simulink model "final_proj_model"  (R2020b)
settings: Solver=ode23tb  StartTime=0  StopTime=365*24*60*60  RelTol=1e-4  EnableMultiTasking=on
StartFcn:
  | tic
StopFcn:
  | toc
values from neighbouring files (symbols this model uses):
  BP1 = [1:24]'    [Build_LoadProfile_Datasets.m]    (also in LoadProfile_Datasets.mat = [1 2 3 4 5 6 7 8 9 10 11 12 ... (24 elements, 24x1)])
  BP2 = [1:3]    [Build_LoadProfile_Datasets.m]    (also in LoadProfile_Datasets.mat = [1 2 3])
  BP3 = [1:2]    [Build_LoadProfile_Datasets.m]    (also in LoadProfile_Datasets.mat = [1 2])
  LoadProfile_Data = [1 2 3 4 5 6 7 8 9 10 11 12 ... (144 elements, 24x3x2)]    [LoadProfile_Datasets.mat]
undefined symbols (not defined in the file or in its folder): A, B, C, D1, Dd, Delta, j, StationData
libraries: powerlib x43, simulink x10, powerlib_meascontrol x8
(part 2 of 2)

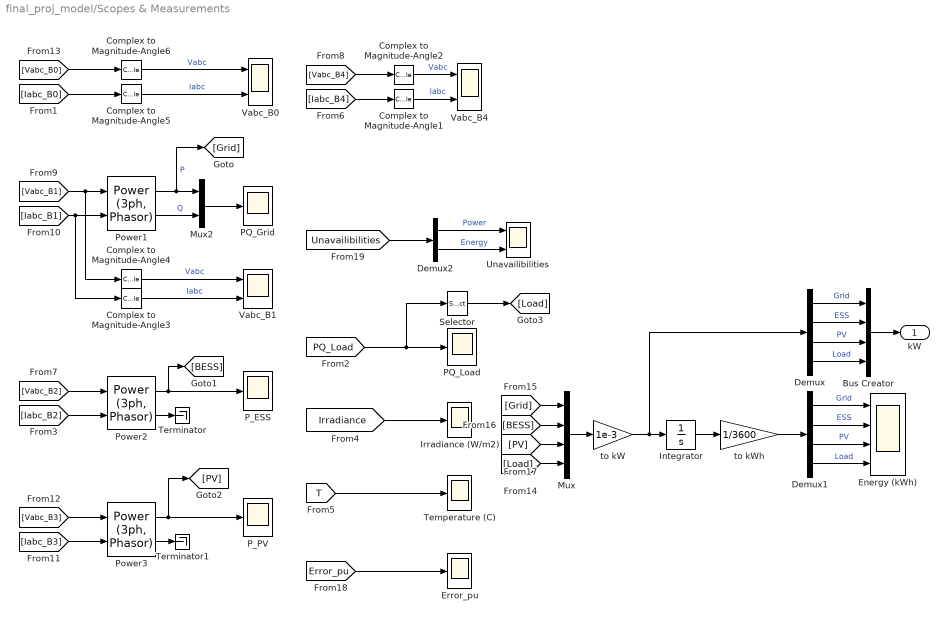
== system final_proj_model/Scopes & Measurements ==
  Bus Creator : BusCreator  Inputs=4
  Complex to Magnitude-Angle{1..6} (6 alike) : ComplexToMagnitudeAngle  Output=Magnitude
  Demux : Demux
  Demux1 : Demux
  Demux2 : Demux  Outputs=2
  Energy (kWh) : Scope  NumInputPorts=4
  Error_pu : Scope
  Integrator : Integrator
  Irradiance (W/m2) : Scope
  Mux : Mux
  Mux2 : Mux  Inputs=2
  PQ_Grid : Scope
  PQ_Load : Scope
  P_ESS : Scope
  P_PV : Scope
  Power1 : powerlib_meascontrol/Measurements/Power (3ph, Phasor)
      settings: SourceProductBaseCode=PS
  Power2 : powerlib_meascontrol/Measurements/Power (3ph, Phasor)
      settings: SourceProductBaseCode=PS
  Power3 : powerlib_meascontrol/Measurements/Power (3ph, Phasor)
      settings: SourceProductBaseCode=PS
  Selector : Selector  InputPortWidth=2  IndexOptions=Index vector (dialog)  Indices=[1]  OutputSizes=1
  Temperature (C) : Scope
  Terminator : Terminator
  Terminator1 : Terminator
  Unavailibilities : Scope  NumInputPorts=2
  Vabc_B0 : Scope  NumInputPorts=2
  Vabc_B1 : Scope  NumInputPorts=2
  Vabc_B4 : Scope  NumInputPorts=2
  to kW : Gain  Gain=1e-3
  to kWh : Gain  Gain=1/3600
  kW : Outport
  wires:
  [Iabc_B1] -> Complex to Magnitude-Angle3/1, Power1/2
  [Vabc_B1] -> Complex to Magnitude-Angle4/1, Power1/1
  Power1/1 -> [Grid], Mux2/1  "P"
  Power1/2 -> Mux2/2  "Q"
  [Iabc_B2] -> Power2/2
  [Vabc_B2] -> Power2/1
  Power2/1 -> P_ESS/1, [BESS]
  [Iabc_B3] -> Power3/2
  [Vabc_B3] -> Power3/1
  Power3/1 -> P_PV/1, [PV]
  Mux2/1 -> PQ_Grid/1
  Complex to Magnitude-Angle4/1 -> Vabc_B1/1  "Vabc"
  Complex to Magnitude-Angle3/1 -> Vabc_B1/2  "Iabc"
  Power2/2 -> Terminator/1
  Power3/2 -> Terminator1/1
  Integrator/1 -> to kWh/1
  Selector/1 -> [Load]
  Bus Creator/1 -> kW/1
  [Grid] -> Mux/1
  [PV] -> Mux/3
  [BESS] -> Mux/2
  [Load] -> Mux/4
  Mux/1 -> to kW/1
  to kW/1 -> Demux/1, Integrator/1
  to kWh/1 -> Demux1/1
  Demux/1 -> Bus Creator/1  "Grid"
  Demux/2 -> Bus Creator/2  "ESS"
  Demux/3 -> Bus Creator/3  "PV"
  Demux/4 -> Bus Creator/4  "Load"
  Demux1/1 -> Energy (kWh)/1  "Grid"
  Demux1/2 -> Energy (kWh)/2  "ESS"
  Demux1/3 -> Energy (kWh)/3  "PV"
  Demux1/4 -> Energy (kWh)/4  "Load"
  [Irradiance] -> Irradiance (W/m2)/1
  [T] -> Temperature (C)/1
  Complex to Magnitude-Angle2/1 -> Vabc_B4/1  "Vabc"
  Complex to Magnitude-Angle1/1 -> Vabc_B4/2  "Iabc"
  [Vabc_B4] -> Complex to Magnitude-Angle2/1
  [Iabc_B4] -> Complex to Magnitude-Angle1/1
  Complex to Magnitude-Angle6/1 -> Vabc_B0/1  "Vabc"
  Complex to Magnitude-Angle5/1 -> Vabc_B0/2  "Iabc"
  [Vabc_B0] -> Complex to Magnitude-Angle6/1
  [Iabc_B0] -> Complex to Magnitude-Angle5/1
  [PQ_Load] -> Selector/1, PQ_Load/1
  [Error_pu] -> Error_pu/1
  [Unavailibilities] -> Demux2/1
  Demux2/1 -> Unavailibilities/1  "Power"
  Demux2/2 -> Unavailibilities/2  "Energy"

== system final_proj_model/Subsystem ==
  Com : Inport
  Fault A : powerlib/Elements/Breaker  InitialState=0  SwitchingTimes=[1e9 1e9+1]  External=on  BreakerResistance=1e-3  SnubberResistance=1e6  SnubberCapacitance=inf  Measurements=None  MoreParameters=off  NoBreakLoop=off
  Fault A1 : powerlib/Elements/Breaker  InitialState=0  SwitchingTimes=[1e9 1e9+1]  External=on  BreakerResistance=1e-3  SnubberResistance=1e6  SnubberCapacitance=inf  Measurements=None  MoreParameters=off  NoBreakLoop=off
  Fault A2 : powerlib/Elements/Breaker  InitialState=0  SwitchingTimes=[1e9 1e9+1]  External=on  BreakerResistance=1e-3  SnubberResistance=1e6  SnubberCapacitance=inf  Measurements=None  MoreParameters=off  NoBreakLoop=off
  a : PMIOPort  Side=Right
  A : PMIOPort  Port=2  Side=Left
  b : PMIOPort  Port=3  Side=Right
  B : PMIOPort  Port=4  Side=Left
  c : PMIOPort  Port=5  Side=Right
  C : PMIOPort  Port=6  Side=Left
  wires:
  Com/1 -> Fault A2/1, Fault A1/1, Fault A/1
  connections:
  Fault A1/RConn1 -- b/RConn1
  Fault A1/LConn1 -- B/RConn1
  Fault A/LConn1 -- A/RConn1
  Fault A2/LConn1 -- C/RConn1
  Fault A/RConn1 -- a/RConn1
  Fault A2/RConn1 -- c/RConn1

== system final_proj_model/TMY3 Data ==
  note: The Irradiance table data are stored in the .mat file StationData_NEW.
      | This file is loaded at  mask initialization.
  note: TMY3 (Typical Meterological Year) files have been produced by NREL's
      | Electric Systems Center under the Solar Resource Characterization Project,
      | which is funded and monitored by the U.S. Department of Energy's Energy
      |  Efficiency and Renewable Energy Office.
  note: National Renewable Energy Laboratory
      | 1617 Cole Boulevard, Golden, Colorado 80401-3393
      | 303-275-3000  www.nrel.gov
  note: Reference: Users Manual for TMY3 Data Sets
      | S. Wilcox and W. Marion
  note: Definition:
      |
      | Global horizontal irradiance, Watt-hour per square meter (Wh/m2)
      | Total amount of direct and diffuse solar radiation received on a
      | horizontal surface during the 60-minute period ending at the timestamp.
      |
      | Diffuse horizontal irradiance, Watt-hour per square meter (Wh/m2)
      | Amount of solar radiation received from the sky (excluding the solar disk)
      | on a horizontal surface during the 60-minute period ending at the timestamp.
      |
      | Direct normal irradiance, Watt-hour per square meter (Wh/m2)
      | Amount of solar radiation (modeled) received in a collimated beam on a surface
      | normal to the sun during the 60-minute period ending at the timestamp.
  1-D Lookup IRRADIANCE Table : Lookup_n-D  NumberOfTableDimensions=1  BreakpointsForDimension1=[1:size(StationData(Index).Temperature,1)]  Table=IrradianceTable  InterpMethod=Flat  InternalRulePriority=Speed  RndMeth=Simplest  InputSameDT=on
  1-D Lookup TEMPERATURE (C) Table : Lookup_n-D  NumberOfTableDimensions=1  BreakpointsForDimension1=[1:size(StationData(Index).Temperature,1)]  Table=StationData(Index).Temperature  InterpMethod=Flat  InternalRulePriority=Speed  RndMeth=Simplest  InputSameDT=on
  1-min Filter : TransferFcn  Denominator=[60 1]
  Add : Sum
  Clock : Clock
  Constant : Constant
  Second-->Hour : Gain  Gain=1/(60*60)
  efficiency : Gain  Gain=Efficiency/100
  m2 : Gain  Gain=TotalArea
  P : Outport
  tag scope: Irradiance=global, T=global
  wires:
  m2/1 -> efficiency/1
  1-D Lookup IRRADIANCE Table/1 -> 1-min Filter/1
  Clock/1 -> Second-->Hour/1
  1-D Lookup TEMPERATURE (C) Table/1 -> [T]
  1-min Filter/1 -> [Irradiance], m2/1
  efficiency/1 -> P/1
  Constant/1 -> Add/2
  Second-->Hour/1 -> Add/1
  Add/1 -> 1-D Lookup TEMPERATURE (C) Table/1, 1-D Lookup IRRADIANCE Table/1  "Hour of the year"

== system final_proj_model/Day Of The Year/Counter ==
  Enable : EnablePort
  Add : Sum
  Constant : Constant
  Memory : Memory
  Out1 : Outport
  wires:
  Add/1 -> Out1/1, Memory/1
  Memory/1 -> Add/1
  Constant/1 -> Add/2

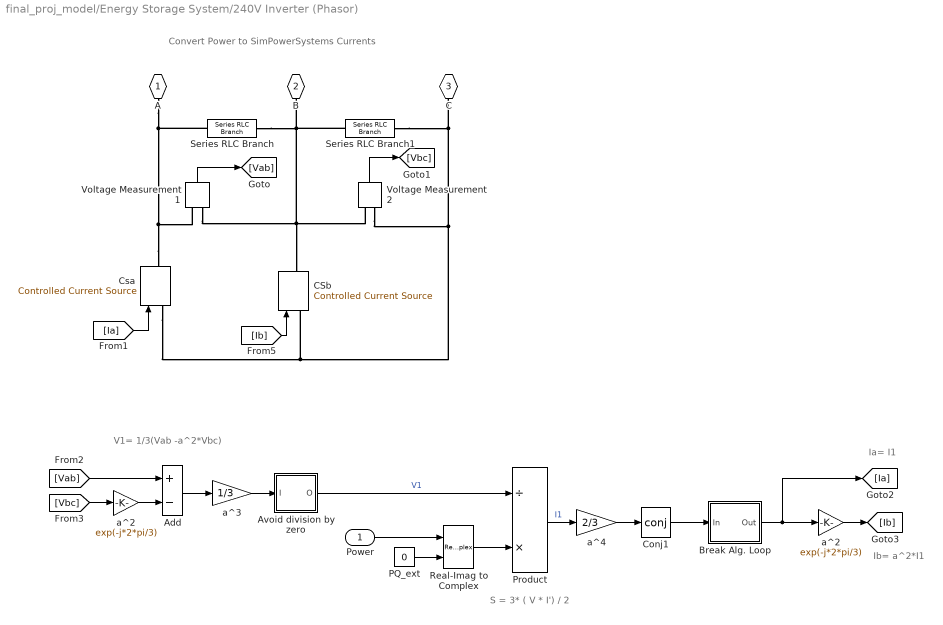
== system final_proj_model/Energy Storage System/240V Inverter (Phasor) ==
  note: V1= 1/3(Vab -a^2*Vbc)
  note: S = 3* ( V * I') / 2
  note: Ia= I1
  note: Ib= a^2*I1
  note: Convert Power to SimPowerSystems Currents
  Power : Inport
  Add : Sum  Inputs=+-
  Avoid division by zero : Subsystem
  "Break Alg. Loop " : Subsystem
  CSb : powerlib/Electrical Sources/Controlled Current Source  Initialize=off  Source_Type=AC  Amplitude=0  Phase=0  Frequency=0  Measurements=None
  Conj1 : Math  Operator=conj  SignedPower=on  SaturateOnIntegerOverflow=on
  Csa : powerlib/Electrical Sources/Controlled Current Source  Initialize=off  Source_Type=AC  Amplitude=0  Phase=0  Frequency=0  Measurements=None
  PQ_ext : Constant  Value=0
  Product : Product  Inputs=/*  InputSameDT=on  SaturateOnIntegerOverflow=on  OutDataTypeStr=Inherit: Same as first input
  Real-Imag to Complex : RealImagToComplex
  Series RLC Branch : powerlib/Elements/Series RLC Branch  LConnTagsString=__new0  RConnTagsString=__new0  BranchType=R  Resistance=1e6  Inductance=1e-3  SetiL0=off  InitialCurrent=0  Capacitance=1e-6  Setx0=off  InitialVoltage=0  Measurements=None
  Series RLC Branch1 : powerlib/Elements/Series RLC Branch  LConnTagsString=__new0  RConnTagsString=__new0  BranchType=R  Resistance=1e6  Inductance=1e-3  SetiL0=off  InitialCurrent=0  Capacitance=1e-6  Setx0=off  InitialVoltage=0  Measurements=None
  Voltage Measurement1 : powerlib/Measurements/Voltage Measurement  PhasorSimulation=on  OutputType=Complex  PSBequivalent=0
  Voltage Measurement2 : powerlib/Measurements/Voltage Measurement  PhasorSimulation=on  OutputType=Complex  PSBequivalent=0
  a^2 : Gain  Gain=exp(-j*2*pi/3)  SaturateOnIntegerOverflow=on  OutDataTypeStr=Inherit: Same as input  ParamDataTypeStr=Inherit: Same as input
  "a^2 " : Gain  Gain=exp(-j*2*pi/3)  SaturateOnIntegerOverflow=on  OutDataTypeStr=Inherit: Same as input  ParamDataTypeStr=Inherit: Same as input
  a^3 : Gain  Gain=1/3  SaturateOnIntegerOverflow=on  OutDataTypeStr=Inherit: Same as input  ParamDataTypeStr=Inherit: Same as input
  a^4 : Gain  Gain=2/3  SaturateOnIntegerOverflow=on  OutDataTypeStr=Inherit: Same as input  ParamDataTypeStr=Inherit: Same as input
  A : PMIOPort  Tag=PMCPort  Side=Right
  B : PMIOPort  Tag=PMCPort  Port=2  Side=Right
  C : PMIOPort  Tag=PMCPort  Port=3  Side=Right
  wires:
  Power/1 -> Real-Imag to Complex/1
  Real-Imag to Complex/1 -> Product/2
  Product/1 -> a^4/1  "I1"
  PQ_ext/1 -> Real-Imag to Complex/2
  a^2/1 -> [Ib]
  Avoid division by zero/1(O) -> Product/1  "V1"
  Conj1/1 -> "Break Alg. Loop "/1(In)
  a^3/1 -> Avoid division by zero/1(I)
  Add/1 -> a^3/1
  [Vab] -> Add/1
  [Vbc] -> "a^2 "/1
  "a^2 "/1 -> Add/2
  a^4/1 -> Conj1/1
  "Break Alg. Loop "/1(Out) -> [Ia], a^2/1
  [Ib] -> CSb/1
  [Ia] -> Csa/1
  Voltage Measurement2/1 -> [Vbc]
  Voltage Measurement1/1 -> [Vab]
  connections:
  Series RLC Branch/RConn1 -- B/RConn1 -- Series RLC Branch1/LConn1 -- CSb/RConn1 -- Voltage Measurement1/LConn2 -- Voltage Measurement2/LConn1
  Series RLC Branch1/RConn1 -- C/RConn1 -- Csa/LConn1 -- CSb/LConn1 -- Voltage Measurement2/LConn2
  Csa/RConn1 -- A/RConn1 -- Series RLC Branch/LConn1 -- Voltage Measurement1/LConn1

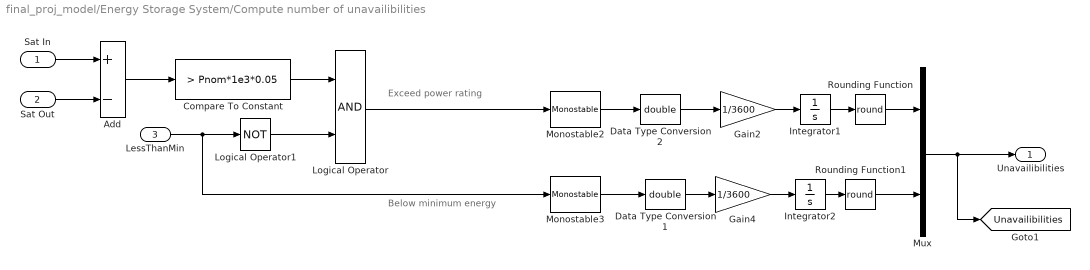
== system final_proj_model/Energy Storage System/Compute number of unavailibilities ==
  note: Exceed power rating
  note: Below minimum energy
  Sat In : Inport
  Sat Out : Inport  Port=2
  LessThanMin : Inport  Port=3
  Add : Sum  Inputs=+-
  Compare To Constant : simulink/Logic and Bit Operations/Compare To Constant  relop=>  const=Pnom*1e3*0.05  OutDataTypeStr=uint8
  Data Type Conversion1 : DataTypeConversion  OutDataTypeStr=double
  Data Type Conversion2 : DataTypeConversion  OutDataTypeStr=double
  Gain2 : Gain  Gain=1/3600
  Gain4 : Gain  Gain=1/3600
  Integrator1 : Integrator
  Integrator2 : Integrator
  Logical Operator : Logic  AllPortsSameDT=off  OutDataTypeStr=boolean
  Logical Operator1 : Logic  Operator=NOT  AllPortsSameDT=off  OutDataTypeStr=boolean
  Monostable2 : powerlib_meascontrol/Logic/Monostable  EdgeDetect=Rising  PulseDuration=3600  ic=0  Ts=0
      settings: SourceProductBaseCode=PS
  Monostable3 : powerlib_meascontrol/Logic/Monostable  EdgeDetect=Rising  PulseDuration=3600  ic=0  Ts=0
      settings: SourceProductBaseCode=PS
  Mux : Mux  Inputs=2
  Rounding Function : Rounding  Operator=round
  Rounding Function1 : Rounding  Operator=round
  Unavailibilities : Outport
  tag scope: Unavailibilities=global
  wires:
  Add/1 -> Compare To Constant/1
  Monostable3/1 -> Data Type Conversion1/1
  Monostable2/1 -> Data Type Conversion2/1
  Data Type Conversion1/1 -> Gain4/1
  Compare To Constant/1 -> Logical Operator/1
  LessThanMin/1 -> Monostable3/1, Logical Operator1/1
  Logical Operator1/1 -> Logical Operator/2
  Data Type Conversion2/1 -> Gain2/1
  Integrator1/1 -> Rounding Function/1
  Integrator2/1 -> Rounding Function1/1
  Rounding Function/1 -> Mux/1
  Rounding Function1/1 -> Mux/2
  Mux/1 -> Unavailibilities/1, [Unavailibilities]
  Logical Operator/1 -> Monostable2/1
  Gain2/1 -> Integrator1/1
  Gain4/1 -> Integrator2/1
  Sat In/1 -> Add/1
  Sat Out/1 -> Add/2

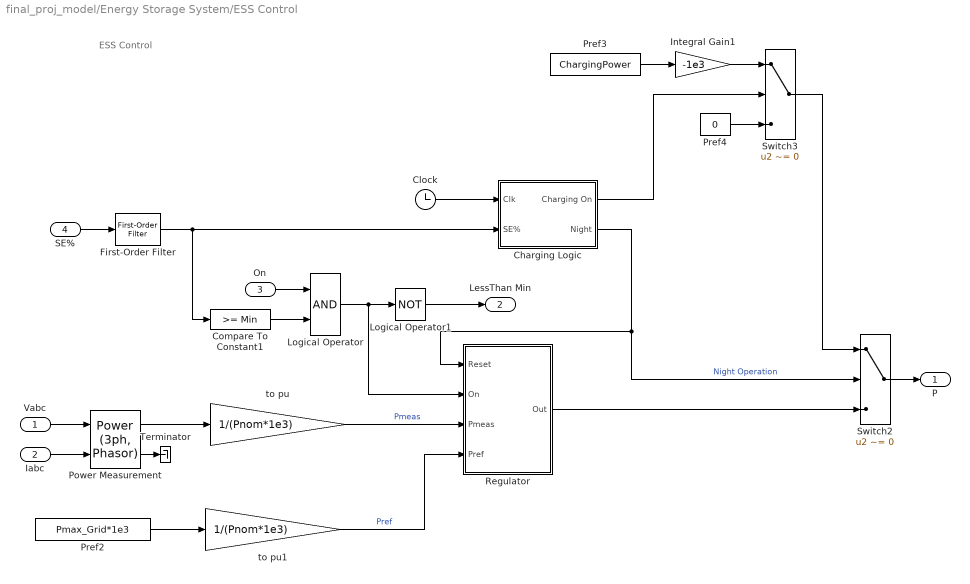
== system final_proj_model/Energy Storage System/ESS Control ==
  note: ESS Control
  Vabc : Inport
  Iabc : Inport  Port=2
  On : Inport  Port=3
  SE% : Inport  Port=4
  Charging Logic : Subsystem
  Clock : Clock
  Compare To Constant1 : simulink/Logic and Bit Operations/Compare To Constant  relop=>=  const=Min  OutDataTypeStr=boolean
  First-Order Filter : powerlib_meascontrol/Filters/First-Order Filter  FilterType=Lowpass  Tc=1  Ts=0  Initialize=on  Vac_Init=[0, 0, 60]  Vdc_Init=Max  PlotResponse=off  FreqRange="[0,  200,  1]"
  Integral Gain1 : Gain  Gain=-1e3
  Logical Operator : Logic  AllPortsSameDT=off  OutDataTypeStr=boolean
  Logical Operator1 : Logic  Operator=NOT  AllPortsSameDT=off  OutDataTypeStr=boolean
  Power Measurement : powerlib_meascontrol/Measurements/Power (3ph, Phasor)
      settings: SourceProductBaseCode=PS
  Pref2 : Constant  Value=Pmax_Grid*1e3
  Pref3 : Constant  Value=ChargingPower
  Pref4 : Constant  Value=0
  Regulator : Subsystem
  Switch2 : Switch  Criteria=u2 ~= 0  Threshold=0.5
  Switch3 : Switch  Criteria=u2 ~= 0  Threshold=0.5
  Terminator : Terminator
  to pu : Gain  Gain=1/(Pnom*1e3)
  to pu1 : Gain  Gain=1/(Pnom*1e3)
  P : Outport  OutputWhenDisabled=reset  InitialOutput=0
  LessThan Min : Outport  Port=2  OutputWhenDisabled=reset  InitialOutput=0
  wires:
  Power Measurement/2 -> Terminator/1
  Vabc/1 -> Power Measurement/1
  Iabc/1 -> Power Measurement/2
  Power Measurement/1 -> to pu/1
  Compare To Constant1/1 -> Logical Operator/2
  SE%/1 -> First-Order Filter/1
  Switch2/1 -> P/1
  Pref3/1 -> Integral Gain1/1
  On/1 -> Logical Operator/1
  Clock/1 -> Charging Logic/1(Clk)
  First-Order Filter/1 -> Compare To Constant1/1, Charging Logic/2(SE%)
  Logical Operator/1 -> Regulator/2(On), Logical Operator1/1
  Pref2/1 -> to pu1/1
  Logical Operator1/1 -> LessThan Min/1
  Integral Gain1/1 -> Switch3/1
  Pref4/1 -> Switch3/3
  Switch3/1 -> Switch2/1
  Charging Logic/2(Night) -> Regulator/1(Reset), Switch2/2  "Night Operation"
  Charging Logic/1(Charging On) -> Switch3/2
  to pu/1 -> Regulator/3(Pmeas)  "Pmeas"
  to pu1/1 -> Regulator/4(Pref)  "Pref"
  Regulator/1(Out) -> Switch2/3

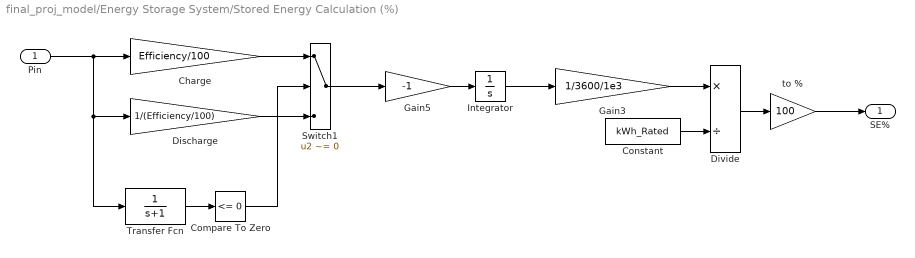
== system final_proj_model/Energy Storage System/Stored Energy Calculation (%) ==
  Pin : Inport
  Charge : Gain  Gain=Efficiency/100
  Compare To Zero : simulink/Logic and Bit Operations/Compare To Zero  relop=<=  OutDataTypeStr=boolean
  Constant : Constant  Value=kWh_Rated
  Discharge : Gain  Gain=1/(Efficiency/100)
  Divide : Product  Inputs=*/
  Gain3 : Gain  Gain=1/3600/1e3
  Gain5 : Gain  Gain=-1
  Integrator : Integrator  InitialCondition=(Initial_kWh_pc/100)*kWh_Rated*3600*1e3
  Switch1 : Switch  Criteria=u2 ~= 0
  Transfer Fcn : TransferFcn  Denominator=[1 1]
  to % : Gain  Gain=100
  SE% : Outport
  wires:
  Pin/1 -> Charge/1, Discharge/1, Transfer Fcn/1
  Integrator/1 -> Gain3/1
  Compare To Zero/1 -> Switch1/2
  Divide/1 -> to %/1
  Charge/1 -> Switch1/1
  Constant/1 -> Divide/2
  Gain3/1 -> Divide/1
  Switch1/1 -> Gain5/1
  Transfer Fcn/1 -> Compare To Zero/1
  to %/1 -> SE%/1
  Gain5/1 -> Integrator/1
  Discharge/1 -> Switch1/3

== system final_proj_model/PV Farm/Avoid division by zero ==
  I : Inport
  Complex to Magnitude-Angle : ComplexToMagnitudeAngle
  Magnitude-Angle to Complex : MagnitudeAngleToComplex
  Saturation1 : Saturate  UpperLimit=inf  LowerLimit=1e-6
  O : Outport
  wires:
  Complex to Magnitude-Angle/2 -> Magnitude-Angle to Complex/2
  Magnitude-Angle to Complex/1 -> O/1
  Complex to Magnitude-Angle/1 -> Saturation1/1
  Saturation1/1 -> Magnitude-Angle to Complex/1
  I/1 -> Complex to Magnitude-Angle/1

== system final_proj_model/PV Farm/Break Alg. Loop  ==
  In : Inport
  Complex to Real-Imag : ComplexToRealImag
  Real-Imag to Complex : RealImagToComplex
  imag : Subsystem  mask(Transfer Function with Initial Outputs){N=[1], D=[1  1], Y0=0, U0=0}
      mask prompts: N "Numerator:"; D "Denominator:"; Y0 "Initial output:"; U0 "Initial input:"
      mask help: Vector expressions for numerator, and denominator. Coefficients are in descending powers of s.
      mask init:
      | [A,B,C,Dd]=tf2ss(N,D);if (isempty(Y0));[m,n]=size(A);X0=zeros(1,m); end; if (isempty(U0));[m,p]=size(B);U0=zeros(1,p);end;X0=getxo(A,B,C,Dd,U0,Y0,0);
      mask Help: Specify the initial output for the transfer function.  An optimization routine attempts to determine the appropriate initial states so that the specified initial output is achieved.  For more details, see the m-file getxo.m
      mask Display: dpoly(N,D,'s')
  real : Subsystem  mask(Transfer Function with Initial Outputs){N=[1], D=[1  1], Y0=0, U0=0}
      mask prompts: N "Numerator:"; D "Denominator:"; Y0 "Initial output:"; U0 "Initial input:"
      mask help: Vector expressions for numerator, and denominator. Coefficients are in descending powers of s.
      mask init:
      | [A,B,C,Dd]=tf2ss(N,D);if (isempty(Y0));[m,n]=size(A);X0=zeros(1,m); end; if (isempty(U0));[m,p]=size(B);U0=zeros(1,p);end;X0=getxo(A,B,C,Dd,U0,Y0,0);
      mask Help: Specify the initial output for the transfer function.  An optimization routine attempts to determine the appropriate initial states so that the specified initial output is achieved.  For more details, see the m-file getxo.m
      mask Display: dpoly(N,D,'s')
  Out : Outport
  wires:
  imag/1(Out1) -> Real-Imag to Complex/2
  Complex to Real-Imag/2 -> imag/1(In1)
  real/1(Out1) -> Real-Imag to Complex/1
  Complex to Real-Imag/1 -> real/1(In1)
  Real-Imag to Complex/1 -> Out/1
  In/1 -> Complex to Real-Imag/1

== system final_proj_model/Residential Load/Determine Season ==
  note: Winter = First 3 months + last 3 months
  Clk : Inport
  3 months in seconds : simulink/Logic and Bit Operations/Compare To Constant  relop=>=  const=(8760*1/4)*60*60  OutDataTypeStr=boolean
  9 months in seconds : simulink/Logic and Bit Operations/Compare To Constant  relop=<  const=(8760*3/4)*60*60  OutDataTypeStr=boolean
  Logical Operator : Logic  AllPortsSameDT=off  OutDataTypeStr=boolean
  Summer : Constant  Value=2
  Switch : Switch  Criteria=u2 ~= 0
  Winter : Constant  Value=3
  Season : Outport
  wires:
  Switch/1 -> Season/1
  Clk/1 -> 9 months in seconds/1, 3 months in seconds/1
  Logical Operator/1 -> Switch/2
  Winter/1 -> Switch/3
  Summer/1 -> Switch/1
  9 months in seconds/1 -> Logical Operator/2
  3 months in seconds/1 -> Logical Operator/1

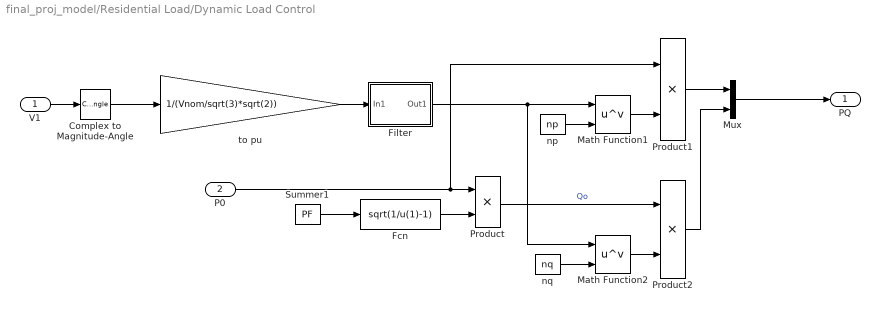
== system final_proj_model/Residential Load/Dynamic Load Control ==
  V1 : Inport
  P0 : Inport  Port=2
  Complex to Magnitude-Angle : ComplexToMagnitudeAngle  Output=Magnitude
  Fcn : Fcn  Expr=sqrt(1/u(1)-1)
  Filter : Subsystem  mask(Transfer Function with Initial Outputs){N=[1], D=[1  1], Y0=0, U0=0}
      mask prompts: N "Numerator:"; D "Denominator:"; Y0 "Initial output:"; U0 "Initial input:"
      mask help: Vector expressions for numerator, and denominator. Coefficients are in descending powers of s.
      mask init:
      | [A,B,C,Dd]=tf2ss(N,D);if (isempty(Y0));[m,n]=size(A);X0=zeros(1,m); end; if (isempty(U0));[m,p]=size(B);U0=zeros(1,p);end;X0=getxo(A,B,C,Dd,U0,Y0,0);
      mask Help: Specify the initial output for the transfer function.  An optimization routine attempts to determine the appropriate initial states so that the specified initial output is achieved.  For more details, see the m-file getxo.m
      mask Display: dpoly(N,D,'s')
  Math Function1 : Math  Operator=pow  SignedPower=on  SaturateOnIntegerOverflow=on
  Math Function2 : Math  Operator=pow  SignedPower=on  SaturateOnIntegerOverflow=on
  Mux : Mux  Inputs=2
  Product : Product
  Product1 : Product
  Product2 : Product
  Summer1 : Constant  Value=PF
  np : Constant  Value=np
  nq : Constant  Value=nq
  to pu : Gain  Gain=1/(Vnom/sqrt(3)*sqrt(2))  SaturateOnIntegerOverflow=on  OutDataTypeStr=Inherit: Same as input  ParamDataTypeStr=Inherit: Same as input
  PQ : Outport
  wires:
  Summer1/1 -> Fcn/1
  P0/1 -> Product1/1, Product/1
  Complex to Magnitude-Angle/1 -> to pu/1
  to pu/1 -> Filter/1(In1)
  Fcn/1 -> Product/2
  Product1/1 -> Mux/1
  Product2/1 -> Mux/2
  Mux/1 -> PQ/1
  Filter/1(Out1) -> Math Function2/1, Math Function1/1
  Math Function1/1 -> Product1/2
  Product/1 -> Product2/1  "Qo"
  Math Function2/1 -> Product2/2
  nq/1 -> Math Function2/2
  np/1 -> Math Function1/2
  V1/1 -> Complex to Magnitude-Angle/1

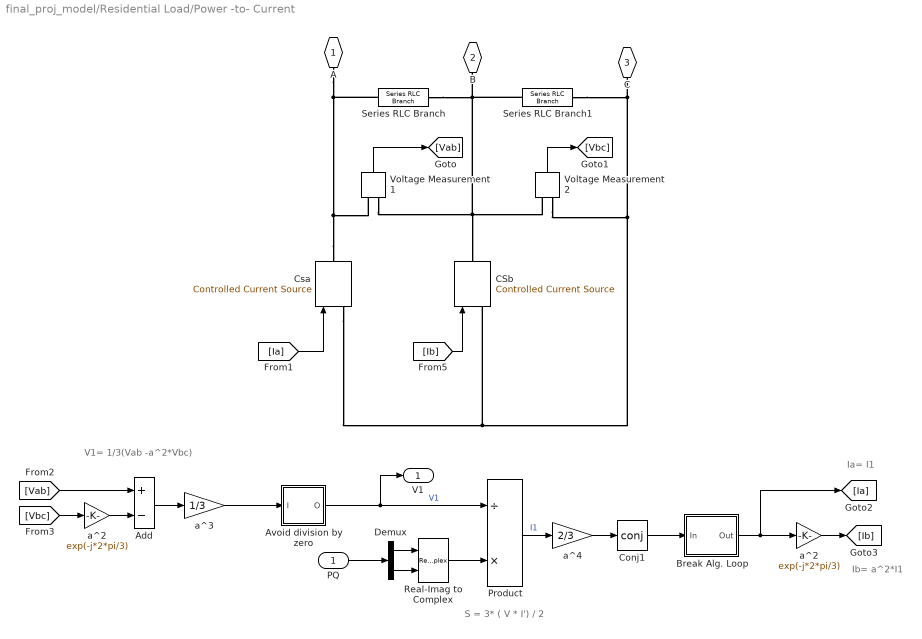
== system final_proj_model/Residential Load/Power -to- Current ==
  note: V1= 1/3(Vab -a^2*Vbc)
  note: S = 3* ( V * I') / 2
  note: Ia= I1
  note: Ib= a^2*I1
  PQ : Inport
  Add : Sum  Inputs=+-
  Avoid division by zero : Subsystem
  "Break Alg. Loop " : Subsystem
  CSb : powerlib/Electrical Sources/Controlled Current Source  Initialize=off  Source_Type=AC  Amplitude=0  Phase=0  Frequency=0  Measurements=None
  Conj1 : Math  Operator=conj  SignedPower=on  SaturateOnIntegerOverflow=on
  Csa : powerlib/Electrical Sources/Controlled Current Source  Initialize=off  Source_Type=AC  Amplitude=0  Phase=0  Frequency=0  Measurements=None
  Demux : Demux  Outputs=2
  Product : Product  Inputs=/*  InputSameDT=on  SaturateOnIntegerOverflow=on  OutDataTypeStr=Inherit: Same as first input
  Real-Imag to Complex : RealImagToComplex
  Series RLC Branch : powerlib/Elements/Series RLC Branch  LConnTagsString=__new0  RConnTagsString=__new0  BranchType=R  Resistance=1e6  Inductance=1e-3  SetiL0=off  InitialCurrent=0  Capacitance=1e-6  Setx0=off  InitialVoltage=0  Measurements=None
  Series RLC Branch1 : powerlib/Elements/Series RLC Branch  LConnTagsString=__new0  RConnTagsString=__new0  BranchType=R  Resistance=1e6  Inductance=1e-3  SetiL0=off  InitialCurrent=0  Capacitance=1e-6  Setx0=off  InitialVoltage=0  Measurements=None
  Voltage Measurement1 : powerlib/Measurements/Voltage Measurement  PhasorSimulation=on  OutputType=Complex  PSBequivalent=0
  Voltage Measurement2 : powerlib/Measurements/Voltage Measurement  PhasorSimulation=on  OutputType=Complex  PSBequivalent=0
  a^2 : Gain  Gain=exp(-j*2*pi/3)  SaturateOnIntegerOverflow=on  OutDataTypeStr=Inherit: Same as input  ParamDataTypeStr=Inherit: Same as input
  "a^2 " : Gain  Gain=exp(-j*2*pi/3)  SaturateOnIntegerOverflow=on  OutDataTypeStr=Inherit: Same as input  ParamDataTypeStr=Inherit: Same as input
  a^3 : Gain  Gain=1/3  SaturateOnIntegerOverflow=on  OutDataTypeStr=Inherit: Same as input  ParamDataTypeStr=Inherit: Same as input
  a^4 : Gain  Gain=2/3  SaturateOnIntegerOverflow=on  OutDataTypeStr=Inherit: Same as input  ParamDataTypeStr=Inherit: Same as input
  A : PMIOPort  Tag=PMCPort  Side=Right
  B : PMIOPort  Tag=PMCPort  Port=2  Side=Right
  C : PMIOPort  Tag=PMCPort  Port=3  Side=Right
  V1 : Outport
  wires:
  Voltage Measurement1/1 -> [Vab]
  Voltage Measurement2/1 -> [Vbc]
  Real-Imag to Complex/1 -> Product/2
  Product/1 -> a^4/1  "I1"
  [Ia] -> Csa/1
  a^2/1 -> [Ib]
  Avoid division by zero/1(O) -> V1/1, Product/1  "V1"
  Conj1/1 -> "Break Alg. Loop "/1(In)
  a^3/1 -> Avoid division by zero/1(I)
  Add/1 -> a^3/1
  [Vab] -> Add/1
  [Vbc] -> "a^2 "/1
  "a^2 "/1 -> Add/2
  a^4/1 -> Conj1/1
  "Break Alg. Loop "/1(Out) -> [Ia], a^2/1
  [Ib] -> CSb/1
  Demux/1 -> Real-Imag to Complex/1
  Demux/2 -> Real-Imag to Complex/2
  PQ/1 -> Demux/1
  connections:
  Csa/RConn1 -- Voltage Measurement1/LConn1 -- Series RLC Branch/LConn1 -- A/RConn1
  C/RConn1 -- Series RLC Branch1/RConn1 -- Csa/LConn1 -- CSb/LConn1 -- Voltage Measurement2/LConn2
  B/RConn1 -- Series RLC Branch/RConn1 -- Series RLC Branch1/LConn1 -- Voltage Measurement2/LConn1 -- Voltage Measurement1/LConn2 -- CSb/RConn1

== system final_proj_model/Energy Storage System/240V Inverter (Phasor)/Avoid division by zero ==
  I : Inport
  Complex to Magnitude-Angle : ComplexToMagnitudeAngle
  Magnitude-Angle to Complex : MagnitudeAngleToComplex
  Saturation1 : Saturate  UpperLimit=inf  LowerLimit=1e-6
  O : Outport
  wires:
  I/1 -> Complex to Magnitude-Angle/1
  Saturation1/1 -> Magnitude-Angle to Complex/1
  Complex to Magnitude-Angle/1 -> Saturation1/1
  Magnitude-Angle to Complex/1 -> O/1
  Complex to Magnitude-Angle/2 -> Magnitude-Angle to Complex/2

== system final_proj_model/Energy Storage System/240V Inverter (Phasor)/Break Alg. Loop  ==
  In : Inport
  Complex to Real-Imag : ComplexToRealImag
  Real-Imag to Complex : RealImagToComplex
  imag : Subsystem  mask(Transfer Function with Initial Outputs){N=[1], D=[1  1], Y0=0, U0=0}
      mask prompts: N "Numerator:"; D "Denominator:"; Y0 "Initial output:"; U0 "Initial input:"
      mask help: Vector expressions for numerator, and denominator. Coefficients are in descending powers of s.
      mask init:
      | [A,B,C,Dd]=tf2ss(N,D);if (isempty(Y0));[m,n]=size(A);X0=zeros(1,m); end; if (isempty(U0));[m,p]=size(B);U0=zeros(1,p);end;X0=getxo(A,B,C,Dd,U0,Y0,0);
      mask Help: Specify the initial output for the transfer function.  An optimization routine attempts to determine the appropriate initial states so that the specified initial output is achieved.  For more details, see the m-file getxo.m
      mask Display: dpoly(N,D,'s')
  real : Subsystem  mask(Transfer Function with Initial Outputs){N=[1], D=[1  1], Y0=0, U0=0}
      mask prompts: N "Numerator:"; D "Denominator:"; Y0 "Initial output:"; U0 "Initial input:"
      mask help: Vector expressions for numerator, and denominator. Coefficients are in descending powers of s.
      mask init:
      | [A,B,C,Dd]=tf2ss(N,D);if (isempty(Y0));[m,n]=size(A);X0=zeros(1,m); end; if (isempty(U0));[m,p]=size(B);U0=zeros(1,p);end;X0=getxo(A,B,C,Dd,U0,Y0,0);
      mask Help: Specify the initial output for the transfer function.  An optimization routine attempts to determine the appropriate initial states so that the specified initial output is achieved.  For more details, see the m-file getxo.m
      mask Display: dpoly(N,D,'s')
  Out : Outport
  wires:
  In/1 -> Complex to Real-Imag/1
  Real-Imag to Complex/1 -> Out/1
  Complex to Real-Imag/1 -> real/1(In1)
  real/1(Out1) -> Real-Imag to Complex/1
  Complex to Real-Imag/2 -> imag/1(In1)
  imag/1(Out1) -> Real-Imag to Complex/2

== system final_proj_model/Energy Storage System/ESS Control/Charging Logic ==
  note: Charging is allowed between midnight and 6 o'clock in the morning if Stored Energy is less than 90 %
  Clk : Inport
  SE% : Inport  Port=2
  1 day in hours : Constant  Value=24
  Compare To Constant : simulink/Logic and Bit Operations/Compare To Constant  relop=<  const=Max  OutDataTypeStr=boolean
  Logical Operator1 : Logic  AllPortsSameDT=off  OutDataTypeStr=boolean
  Math Function : Math  Operator=mod  SignedPower=on  SaturateOnIntegerOverflow=on
  Second-->Hour : Gain  Gain=1/(60*60)
  night : simulink/Logic and Bit Operations/Compare To Constant  relop=<  const=6  OutDataTypeStr=boolean
  Charging On : Outport
  Night : Outport  Port=2
  wires:
  Logical Operator1/1 -> Charging On/1
  Second-->Hour/1 -> Math Function/1
  Math Function/1 -> night/1
  1 day in hours/1 -> Math Function/2
  night/1 -> Night/1, Logical Operator1/1
  SE%/1 -> Compare To Constant/1
  Compare To Constant/1 -> Logical Operator1/2
  Clk/1 -> Second-->Hour/1

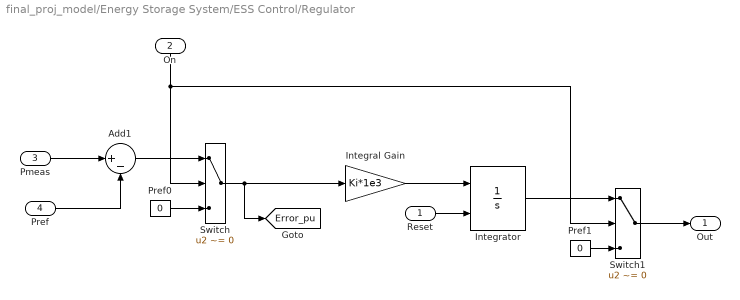
== system final_proj_model/Energy Storage System/ESS Control/Regulator ==
  Reset : Inport
  On : Inport  Port=2
  Pmeas : Inport  Port=3
  Pref : Inport  Port=4
  Add1 : Sum  Inputs=|+-
  Integral Gain : Gain  Gain=Ki*1e3
  Integrator : Integrator  ExternalReset=falling  LimitOutput=on  UpperSaturationLimit=Plimit*1.1  LowerSaturationLimit=0
  Pref0 : Constant  Value=0
  Pref1 : Constant  Value=0
  Switch : Switch  Criteria=u2 ~= 0  Threshold=0.5
  Switch1 : Switch  Criteria=u2 ~= 0  Threshold=0.5
  Out : Outport
  tag scope: Error_pu=global
  wires:
  Reset/1 -> Integrator/2
  On/1 -> Switch1/2, Switch/2
  Pref0/1 -> Switch/3
  Pref1/1 -> Switch1/3
  Integral Gain/1 -> Integrator/1
  Switch/1 -> [Error_pu], Integral Gain/1
  Add1/1 -> Switch/1
  Integrator/1 -> Switch1/1
  Switch1/1 -> Out/1
  Pmeas/1 -> Add1/1
  Pref/1 -> Add1/2

== system final_proj_model/PV Farm/Break Alg. Loop /imag ==
  In1 : Inport
  State Space : StateSpace  A=A  B=B  C=C  D=Dd  InitialCondition=X0
  Out1 : Outport  InitialOutput=0
  wires:
  In1/1 -> State Space/1
  State Space/1 -> Out1/1

== system final_proj_model/PV Farm/Break Alg. Loop /real ==
  In1 : Inport
  State Space : StateSpace  A=A  B=B  C=C  D=Dd  InitialCondition=X0
  Out1 : Outport  InitialOutput=0
  wires:
  In1/1 -> State Space/1
  State Space/1 -> Out1/1

== system final_proj_model/Residential Load/Dynamic Load Control/Filter ==
  In1 : Inport
  State Space : StateSpace  A=A  B=B  C=C  D=Dd  InitialCondition=X0
  Out1 : Outport  InitialOutput=0
  wires:
  State Space/1 -> Out1/1
  In1/1 -> State Space/1

== system final_proj_model/Residential Load/Power -to- Current/Avoid division by zero ==
  I : Inport
  Complex to Magnitude-Angle : ComplexToMagnitudeAngle
  Magnitude-Angle to Complex : MagnitudeAngleToComplex
  Saturation1 : Saturate  UpperLimit=inf  LowerLimit=1e-6
  O : Outport
  wires:
  I/1 -> Complex to Magnitude-Angle/1
  Saturation1/1 -> Magnitude-Angle to Complex/1
  Complex to Magnitude-Angle/1 -> Saturation1/1
  Magnitude-Angle to Complex/1 -> O/1
  Complex to Magnitude-Angle/2 -> Magnitude-Angle to Complex/2

== system final_proj_model/Residential Load/Power -to- Current/Break Alg. Loop  ==
  In : Inport
  Complex to Real-Imag : ComplexToRealImag
  Real-Imag to Complex : RealImagToComplex
  imag : Subsystem  mask(Transfer Function with Initial Outputs){N=[1], D=[1  1], Y0=0, U0=0}
      mask prompts: N "Numerator:"; D "Denominator:"; Y0 "Initial output:"; U0 "Initial input:"
      mask help: Vector expressions for numerator, and denominator. Coefficients are in descending powers of s.
      mask init:
      | [A,B,C,Dd]=tf2ss(N,D);if (isempty(Y0));[m,n]=size(A);X0=zeros(1,m); end; if (isempty(U0));[m,p]=size(B);U0=zeros(1,p);end;X0=getxo(A,B,C,Dd,U0,Y0,0);
      mask Help: Specify the initial output for the transfer function.  An optimization routine attempts to determine the appropriate initial states so that the specified initial output is achieved.  For more details, see the m-file getxo.m
      mask Display: dpoly(N,D,'s')
  real : Subsystem  mask(Transfer Function with Initial Outputs){N=[1], D=[1  1], Y0=0, U0=0}
      mask prompts: N "Numerator:"; D "Denominator:"; Y0 "Initial output:"; U0 "Initial input:"
      mask help: Vector expressions for numerator, and denominator. Coefficients are in descending powers of s.
      mask init:
      | [A,B,C,Dd]=tf2ss(N,D);if (isempty(Y0));[m,n]=size(A);X0=zeros(1,m); end; if (isempty(U0));[m,p]=size(B);U0=zeros(1,p);end;X0=getxo(A,B,C,Dd,U0,Y0,0);
      mask Help: Specify the initial output for the transfer function.  An optimization routine attempts to determine the appropriate initial states so that the specified initial output is achieved.  For more details, see the m-file getxo.m
      mask Display: dpoly(N,D,'s')
  Out : Outport
  wires:
  In/1 -> Complex to Real-Imag/1
  Real-Imag to Complex/1 -> Out/1
  Complex to Real-Imag/1 -> real/1(In1)
  real/1(Out1) -> Real-Imag to Complex/1
  Complex to Real-Imag/2 -> imag/1(In1)
  imag/1(Out1) -> Real-Imag to Complex/2

== system final_proj_model/Energy Storage System/240V Inverter (Phasor)/Break Alg. Loop /imag ==
  In1 : Inport
  State Space : StateSpace  A=A  B=B  C=C  D=Dd  InitialCondition=X0
  Out1 : Outport  InitialOutput=0
  wires:
  State Space/1 -> Out1/1
  In1/1 -> State Space/1

== system final_proj_model/Energy Storage System/240V Inverter (Phasor)/Break Alg. Loop /real ==
  In1 : Inport
  State Space : StateSpace  A=A  B=B  C=C  D=Dd  InitialCondition=X0
  Out1 : Outport  InitialOutput=0
  wires:
  State Space/1 -> Out1/1
  In1/1 -> State Space/1

== system final_proj_model/Residential Load/Power -to- Current/Break Alg. Loop /imag ==
  In1 : Inport
  State Space : StateSpace  A=A  B=B  C=C  D=Dd  InitialCondition=X0
  Out1 : Outport  InitialOutput=0
  wires:
  State Space/1 -> Out1/1
  In1/1 -> State Space/1

== system final_proj_model/Residential Load/Power -to- Current/Break Alg. Loop /real ==
  In1 : Inport
  State Space : StateSpace  A=A  B=B  C=C  D=Dd  InitialCondition=X0
  Out1 : Outport  InitialOutput=0
  wires:
  State Space/1 -> Out1/1
  In1/1 -> State Space/1
